simulink model "TIA"  (R2017b)
settings: Solver=VariableStepAuto  StartTime=0.0  StopTime=inf  RelTol=1e-3
undefined symbols (not defined in the file): sigbuilder_block
(part 1 of 2)
settings Model: PauseTimes=200  NumberOfSteps=10  Creator=matlab01  LastModifiedBy=matlab01

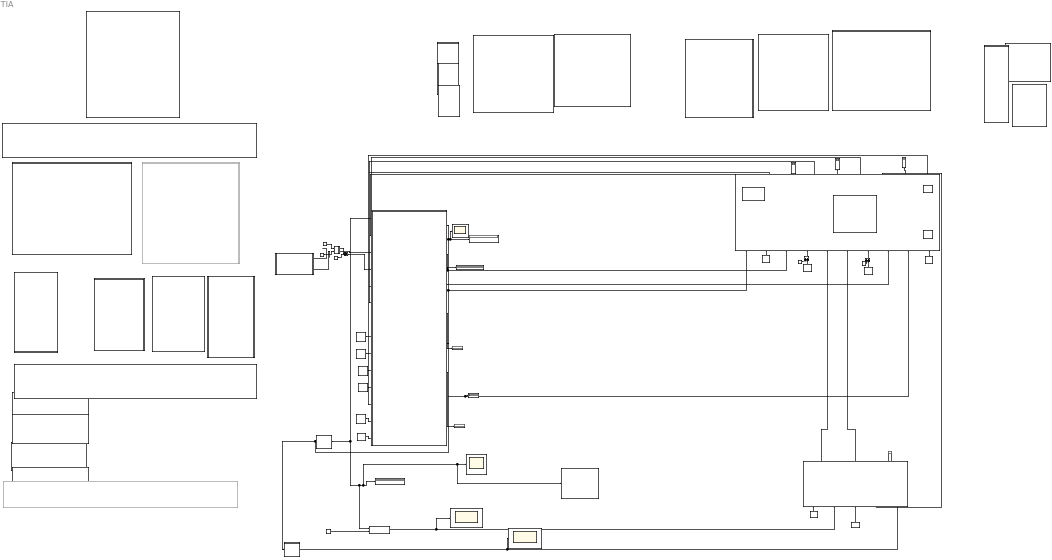
== system TIA ==
  note: Subsystem
  note: Subsystem
  note: User Input Board
  note: Subsystem
  note: Subsystem
  Add : Sum
  Add1 : Sum
  Add2 : Sum
  Bale Pass Sr : Constant  Value=0
  Bale Size Sr : Constant  Value=0
  Baler : Subsystem
  Baler Stopped : Subsystem  DialogController=hmiCreateDDGDialog  IsWebBlock=on  mask(MWDashboardBlock){webBlockId=380f0481-0464-4552-ac21-b39f29efcae4, webBlockType=lamp, ShowInLibBrowser=on, ShowInitialText=on, HMISrcModelName=TIA}
      mask prompts: webBlockType "WebBlock Type"; HMISrcModelName "Source Model"
      mask help: SimulinkHMI:dialogs:LampDialogDesc
      mask Help: helpview([docroot '/mapfiles/simulink.map'], 'hmi_lamp')
      mask Display:
      | if strcmp(get_param(bdroot(gcb),'BlockDiagramType'), 'library')
      |     image([(matlabroot) '/toolbox/simulink/hmi/icons/Lamp.png']);
      | end
  BalerCFG : DisplayBlock  WebBlockId=152  ModelName=TIA  LabelPosition=Hide  ShowInitialText=on  ShowFormattedStrings=off  Format=long  Alignment=Center
  CFG : Display
  Check Box : Checkbox  WebBlockId=154  ModelName=TIA  LabelPosition=Hide  ShowInitialText=off  Checked=on  Label=RearSr_1_Fail
  Check Box1 : Checkbox  WebBlockId=155  ModelName=TIA  LabelPosition=Hide  ShowInitialText=off  Checked=on  Label=RearSr_2_Fail
  Check Box2 : Checkbox  WebBlockId=156  ModelName=TIA  LabelPosition=Hide  ShowInitialText=off  Checked=off  Label=SpeedSr_Fail
  Check Box3 : Checkbox  WebBlockId=157  ModelName=TIA  LabelPosition=Hide  ShowInitialText=off  Checked=off  Label=FrontObstSr_Fail
  Constant : Constant  Value=2
  Constant1 : Constant  Value=2
  Constant2 : Constant  Value=2.7941176470588
  Display{,2,4..6} (5 alike) : Display
  Display3 : DisplayBlock  WebBlockId=163  ModelName=TIA  LabelPosition=Hide  ShowInitialText=on  ShowFormattedStrings=off  Format=long  Alignment=Center
  Display7 : DisplayBlock  WebBlockId=167  ModelName=TIA  LabelPosition=Hide  ShowInitialText=on  ShowFormattedStrings=off  Format=long  Alignment=Center
  DoorStatus : Display
  FinalSysSpeed : Scope
  Front Obstacle : Constant  Value=0
  FrontObstSr : Subsystem
  FrontObstSrFail : Constant  Value=0
  Gauge : Subsystem  DialogController=hmiCreateDDGDialog  IsWebBlock=on  mask(MWDashboardBlock){webBlockId=a8481909-2d34-4551-932e-729d5791eb58, webBlockType=circulargauge, ShowInLibBrowser=on, ShowInitialText=on, HMISrcModelName=TIA}
      mask prompts: webBlockId "WebBlock Id"; webBlockType "WebBlock Type"; HMISrcModelName "Source Model"
      mask help: SimulinkHMI:dialogs:CircularGaugeDialogDesc
      mask Help: helpview([docroot '/mapfiles/simulink.map'], 'hmi_gauge')
      mask Display:
      | if strcmp(get_param(bdroot(gcb),'BlockDiagramType'), 'library')
      |     image([(matlabroot) '/toolbox/simulink/hmi/icons/CircularGauge.png']);
      | end
  Knob : Subsystem  DialogController=hmiCreateDDGDialog  IsWebBlock=on  mask(MWDashboardBlock){webBlockId=44b2cfbf-7851-438f-9afd-65227a1c2716, webBlockType=continuousknob, ShowInLibBrowser=on, ShowInitialText=on, HMISrcModelName=TIA}
      mask prompts: webBlockId "WebBlock Id"; webBlockType "WebBlock Type"; HMISrcModelName "Source Model"
      mask help: SimulinkHMI:dialogs:ContinuousKnobDialogDesc
      mask Help: helpview([docroot '/mapfiles/simulink.map'], 'hmi_knob')
      mask Display:
      | if strcmp(get_param(bdroot(gcb),'BlockDiagramType'), 'library')
      |     image([(matlabroot) '/toolbox/simulink/hmi/icons/ContinuousKnob.png']);
      | end
  Knob1 : Subsystem  DialogController=hmiCreateDDGDialog  IsWebBlock=on  mask(MWDashboardBlock){webBlockId=555d5953-f540-48b0-b281-3241b1506ee0, webBlockType=continuousknob, ShowInLibBrowser=on, ShowInitialText=on, HMISrcModelName=TIA}
      mask prompts: webBlockId "WebBlock Id"; webBlockType "WebBlock Type"; HMISrcModelName "Source Model"
      mask help: SimulinkHMI:dialogs:ContinuousKnobDialogDesc
      mask Help: helpview([docroot '/mapfiles/simulink.map'], 'hmi_knob')
      mask Display:
      | if strcmp(get_param(bdroot(gcb),'BlockDiagramType'), 'library')
      |     image([(matlabroot) '/toolbox/simulink/hmi/icons/ContinuousKnob.png']);
      | end
  Lamp : Subsystem  DialogController=hmiCreateDDGDialog  IsWebBlock=on  mask(MWDashboardBlock){webBlockId=33d9c165-8687-4e0a-bfea-f4d86ec876ec, webBlockType=lamp, ShowInLibBrowser=on, ShowInitialText=on, HMISrcModelName=TIA}
      mask prompts: webBlockType "WebBlock Type"; HMISrcModelName "Source Model"
      mask help: SimulinkHMI:dialogs:LampDialogDesc
      mask Help: helpview([docroot '/mapfiles/simulink.map'], 'hmi_lamp')
      mask Display:
      | if strcmp(get_param(bdroot(gcb),'BlockDiagramType'), 'library')
      |     image([(matlabroot) '/toolbox/simulink/hmi/icons/Lamp.png']);
      | end
  Lamp1 : Subsystem  DialogController=hmiCreateDDGDialog  IsWebBlock=on  mask(MWDashboardBlock){webBlockId=c492ce9b-3337-4b76-9797-8f79f533d9ec, webBlockType=lamp, ShowInLibBrowser=on, ShowInitialText=on, HMISrcModelName=TIA}
      mask prompts: webBlockType "WebBlock Type"; HMISrcModelName "Source Model"
      mask help: SimulinkHMI:dialogs:LampDialogDesc
      mask Help: helpview([docroot '/mapfiles/simulink.map'], 'hmi_lamp')
      mask Display:
      | if strcmp(get_param(bdroot(gcb),'BlockDiagramType'), 'library')
      |     image([(matlabroot) '/toolbox/simulink/hmi/icons/Lamp.png']);
      | end
  Lamp2 : Subsystem  DialogController=hmiCreateDDGDialog  IsWebBlock=on  mask(MWDashboardBlock){webBlockId=4733d592-1260-498b-b033-10984541e09d, webBlockType=lamp, ShowInLibBrowser=on, ShowInitialText=on, HMISrcModelName=TIA}
      mask prompts: webBlockType "WebBlock Type"; HMISrcModelName "Source Model"
      mask help: SimulinkHMI:dialogs:LampDialogDesc
      mask Help: helpview([docroot '/mapfiles/simulink.map'], 'hmi_lamp')
      mask Display:
      | if strcmp(get_param(bdroot(gcb),'BlockDiagramType'), 'library')
      |     image([(matlabroot) '/toolbox/simulink/hmi/icons/Lamp.png']);
      | end
  Lamp3 : Subsystem  DialogController=hmiCreateDDGDialog  IsWebBlock=on  mask(MWDashboardBlock){webBlockId=748ac69b-6fb4-4b5c-9b27-9bec6aca2e03, webBlockType=lamp, ShowInLibBrowser=on, ShowInitialText=on, HMISrcModelName=TIA}
      mask prompts: webBlockType "WebBlock Type"; HMISrcModelName "Source Model"
      mask help: SimulinkHMI:dialogs:LampDialogDesc
      mask Help: helpview([docroot '/mapfiles/simulink.map'], 'hmi_lamp')
      mask Display:
      | if strcmp(get_param(bdroot(gcb),'BlockDiagramType'), 'library')
      |     image([(matlabroot) '/toolbox/simulink/hmi/icons/Lamp.png']);
      | end
  Lamp4 : Subsystem  DialogController=hmiCreateDDGDialog  IsWebBlock=on  mask(MWDashboardBlock){webBlockId=46aeaf17-ce96-4d45-93cb-a6cc3236d1da, webBlockType=lamp, ShowInLibBrowser=on, ShowInitialText=on, HMISrcModelName=TIA}
      mask prompts: webBlockType "WebBlock Type"; HMISrcModelName "Source Model"
      mask help: SimulinkHMI:dialogs:LampDialogDesc
      mask Help: helpview([docroot '/mapfiles/simulink.map'], 'hmi_lamp')
      mask Display:
      | if strcmp(get_param(bdroot(gcb),'BlockDiagramType'), 'library')
      |     image([(matlabroot) '/toolbox/simulink/hmi/icons/Lamp.png']);
      | end
  Lamp5 : Subsystem  DialogController=hmiCreateDDGDialog  IsWebBlock=on  mask(MWDashboardBlock){webBlockId=a14f3337-2fd1-43d0-b24a-5146b7c5b984, webBlockType=lamp, ShowInLibBrowser=on, ShowInitialText=on, HMISrcModelName=TIA}
      mask prompts: webBlockType "WebBlock Type"; HMISrcModelName "Source Model"
      mask help: SimulinkHMI:dialogs:LampDialogDesc
      mask Help: helpview([docroot '/mapfiles/simulink.map'], 'hmi_lamp')
      mask Display:
      | if strcmp(get_param(bdroot(gcb),'BlockDiagramType'), 'library')
      |     image([(matlabroot) '/toolbox/simulink/hmi/icons/Lamp.png']);
      | end
  Lamp6 : Subsystem  DialogController=hmiCreateDDGDialog  IsWebBlock=on  mask(MWDashboardBlock){webBlockId=0c8923f2-3b37-4230-bb87-17ac293e5df4, webBlockType=lamp, ShowInLibBrowser=on, ShowInitialText=on, HMISrcModelName=TIA}
      mask prompts: webBlockType "WebBlock Type"; HMISrcModelName "Source Model"
      mask help: SimulinkHMI:dialogs:LampDialogDesc
      mask Help: helpview([docroot '/mapfiles/simulink.map'], 'hmi_lamp')
      mask Display:
      | if strcmp(get_param(bdroot(gcb),'BlockDiagramType'), 'library')
      |     image([(matlabroot) '/toolbox/simulink/hmi/icons/Lamp.png']);
      | end
  Linear Gauge : Subsystem  DialogController=hmiCreateDDGDialog  IsWebBlock=on  mask(MWDashboardBlock){webBlockId=3991d636-6193-4a79-b88e-7eb4f4bb3acf, webBlockType=lineargauge, ShowInLibBrowser=on, ShowInitialText=on, HMISrcModelName=TIA}
      mask prompts: webBlockId "WebBlock Id"; webBlockType "WebBlock Type"; HMISrcModelName "Source Model"
      mask help: SimulinkHMI:dialogs:LinearGaugeDialogDesc
      mask Help: helpview([docroot '/mapfiles/simulink.map'], 'hmi_linear_gauge')
      mask Display:
      | if strcmp(get_param(bdroot(gcb),'BlockDiagramType'), 'library')
      |     image([(matlabroot) '/toolbox/simulink/hmi/icons/LinearGauge.png']);
      | end
  Need to stop : Display
  Product : Product
  RearDoor : Subsystem  DialogController=hmiCreateDDGDialog  IsWebBlock=on  mask(MWDashboardBlock){webBlockId=b538fc73-89be-495c-b7c3-b8c3e3397391, webBlockType=lamp, ShowInLibBrowser=on, ShowInitialText=on, HMISrcModelName=TIA}
      mask prompts: webBlockType "WebBlock Type"; HMISrcModelName "Source Model"
      mask help: SimulinkHMI:dialogs:LampDialogDesc
      mask Help: helpview([docroot '/mapfiles/simulink.map'], 'hmi_lamp')
      mask Display:
      | if strcmp(get_param(bdroot(gcb),'BlockDiagramType'), 'library')
      |     image([(matlabroot) '/toolbox/simulink/hmi/icons/Lamp.png']);
      | end
  RearObstSr : Subsystem  DialogController=hmiCreateDDGDialog  IsWebBlock=on  mask(MWDashboardBlock){webBlockId=2f04e0dc-cfdf-4b89-b502-650f31ce5fe2, webBlockType=rockerswitch, ShowInLibBrowser=on, ShowInitialText=on, HMISrcModelName=TIA}
      mask prompts: webBlockId "WebBlock Id"; webBlockType "WebBlock Type"; HMISrcModelName "Source Model"
      mask help: SimulinkHMI:dialogs:SwitchDialogDesc
      mask Help: helpview([docroot '/mapfiles/simulink.map'], 'hmi_rocker_switch')
      mask Display:
      | if strcmp(get_param(bdroot(gcb),'BlockDiagramType'), 'library')
      |     image([(matlabroot) '/toolbox/simulink/hmi/icons/RockerSwitch.png']);
      | end
  RearObstSr1 : Subsystem  DialogController=hmiCreateDDGDialog  IsWebBlock=on  mask(MWDashboardBlock){webBlockId=c64d6447-8e55-46e9-b568-5078a23053e9, webBlockType=rockerswitch, ShowInLibBrowser=on, ShowInitialText=on, HMISrcModelName=TIA}
      mask prompts: webBlockId "WebBlock Id"; webBlockType "WebBlock Type"; HMISrcModelName "Source Model"
      mask help: SimulinkHMI:dialogs:SwitchDialogDesc
      mask Help: helpview([docroot '/mapfiles/simulink.map'], 'hmi_rocker_switch')
      mask Display:
      | if strcmp(get_param(bdroot(gcb),'BlockDiagramType'), 'library')
      |     image([(matlabroot) '/toolbox/simulink/hmi/icons/RockerSwitch.png']);
      | end
  RearObstSr2 : Subsystem  DialogController=hmiCreateDDGDialog  IsWebBlock=on  mask(MWDashboardBlock){webBlockId=c4afeddd-f4a6-4f0c-9e01-adb611532535, webBlockType=rockerswitch, ShowInLibBrowser=on, ShowInitialText=on, HMISrcModelName=TIA}
      mask prompts: webBlockId "WebBlock Id"; webBlockType "WebBlock Type"; HMISrcModelName "Source Model"
      mask help: SimulinkHMI:dialogs:SwitchDialogDesc
      mask Help: helpview([docroot '/mapfiles/simulink.map'], 'hmi_rocker_switch')
      mask Display:
      | if strcmp(get_param(bdroot(gcb),'BlockDiagramType'), 'library')
      |     image([(matlabroot) '/toolbox/simulink/hmi/icons/RockerSwitch.png']);
      | end
  RearSr1 : Constant  Value=0
  RearSr2 : Constant  Value=0
  Rotary Switch : Subsystem  DialogController=hmiCreateDDGDialog  IsWebBlock=on  mask(MWDashboardBlock){webBlockId=4718e849-02b3-481c-8935-c4c34f11cecd, webBlockType=discreteknob, ShowInLibBrowser=on, ShowInitialText=on, HMISrcModelName=TIA}
      mask prompts: webBlockId "WebBlock Id"; webBlockType "WebBlock Type"; HMISrcModelName "Source Model"
      mask help: SimulinkHMI:dialogs:DiscreteKnobDialogDesc
      mask Help: helpview([docroot '/mapfiles/simulink.map'], 'hmi_rotary_switch')
      mask Display:
      | model = bdroot(gcb);
      | if strcmp(get_param(model,'BlockDiagramType'), 'library')
      |     image([(matlabroot) '/toolbox/simulink/hmi/icons/DiscreteKnob.png']);
      | end
  Rotary Switch1 : Subsystem  DialogController=hmiCreateDDGDialog  IsWebBlock=on  mask(MWDashboardBlock){webBlockId=f404cd82-44b9-4011-b588-6289506ab41c, webBlockType=discreteknob, ShowInLibBrowser=on, ShowInitialText=on, HMISrcModelName=TIA}
      mask prompts: webBlockId "WebBlock Id"; webBlockType "WebBlock Type"; HMISrcModelName "Source Model"
      mask help: SimulinkHMI:dialogs:DiscreteKnobDialogDesc
      mask Help: helpview([docroot '/mapfiles/simulink.map'], 'hmi_rotary_switch')
      mask Display:
      | model = bdroot(gcb);
      | if strcmp(get_param(model,'BlockDiagramType'), 'library')
      |     image([(matlabroot) '/toolbox/simulink/hmi/icons/DiscreteKnob.png']);
      | end
  Rotary Switch3 : Subsystem  DialogController=hmiCreateDDGDialog  IsWebBlock=on  mask(MWDashboardBlock){webBlockId=10fa69e3-8ad0-4a7e-b427-115ef8b6ee24, webBlockType=discreteknob, ShowInLibBrowser=on, ShowInitialText=on, HMISrcModelName=TIA}
      mask prompts: webBlockId "WebBlock Id"; webBlockType "WebBlock Type"; HMISrcModelName "Source Model"
      mask help: SimulinkHMI:dialogs:DiscreteKnobDialogDesc
      mask Help: helpview([docroot '/mapfiles/simulink.map'], 'hmi_rotary_switch')
      mask Display:
      | model = bdroot(gcb);
      | if strcmp(get_param(model,'BlockDiagramType'), 'library')
      |     image([(matlabroot) '/toolbox/simulink/hmi/icons/DiscreteKnob.png']);
      | end
  Scope : Scope
  SettedSpeed : Display
  Signal Builder : Subsystem  Tag=STV Subsys  LoadFcn=sigbuilder_block('load');  StartFcn=sigbuilder_block('start');  StopFcn=sigbuilder_block('stop');  ClipboardFcn=sigbuilder_block('clipboard');  mask(Sigbuilder block){tuvar=[0:10]}
      mask help: Simulink:masks:SigbuilderBlock_MD
      mask init:
      | if ~strcmp(get_param(bdroot(gcbh),'SimulationStatus'),'stopped') tuvar = sigbuilder_block('maskInit'); end
      settings: CopyFcn=sigbuilder_block('copy');  DeleteFcn=sigbuilder_block('delete');  ModelCloseFcn=sigbuilder_block('modelClose');  PreSaveFcn=sigbuilder_block('preSave');  PauseFcn=sigbuilder_block('pause');  ContinueFcn=sigbuilder_block('continue');  NameChangeFcn=sigbuilder_block('namechange');  OpenFcn=sigbuilder_block('open',[107.25 -48.75 897.75 700.5 ]);  CloseFcn=sigbuilder_block('close');
      mask Display: plot(0, 0, 100, 100,[2, 2, 32, 32, 2], [68, 8, 8, 68, 68],[32, 2], [38, 38], [32, 19, 2],[53, 60, 44], [32, 17, 17, 2],[16, 16, 31, 31]);txt = getActiveGroup(gcbh);text(2, 100, txt,'verticalAlignment', 'top');
  Slider : Subsystem  Commented=on  DialogController=hmiCreateDDGDialog  IsWebBlock=on  mask(MWDashboardBlock){webBlockId=15a6815c-0950-4bd8-89d9-de0febee8296, webBlockType=slider, ShowInLibBrowser=on, ShowInitialText=on, HMISrcModelName=TIA}
      mask prompts: webBlockId "WebBlock Id"; webBlockType "WebBlock Type"; HMISrcModelName "Source Model"
      mask help: SimulinkHMI:dialogs:SliderDialogDesc
      mask Help: helpview([docroot '/mapfiles/simulink.map'], 'hmi_slider')
      mask Display:
      | if strcmp(get_param(bdroot(gcb),'BlockDiagramType'), 'library')
      |     image([(matlabroot) '/toolbox/simulink/hmi/icons/Slider.png']);
      | end
  Slider1 : Subsystem  DialogController=hmiCreateDDGDialog  IsWebBlock=on  mask(MWDashboardBlock){webBlockId=472954f7-77f4-4c52-b158-1c9b312c99f5, webBlockType=slider, ShowInLibBrowser=on, ShowInitialText=on, HMISrcModelName=TIA}
      mask prompts: webBlockId "WebBlock Id"; webBlockType "WebBlock Type"; HMISrcModelName "Source Model"
      mask help: SimulinkHMI:dialogs:SliderDialogDesc
      mask Help: helpview([docroot '/mapfiles/simulink.map'], 'hmi_slider')
      mask Display:
      | if strcmp(get_param(bdroot(gcb),'BlockDiagramType'), 'library')
      |     image([(matlabroot) '/toolbox/simulink/hmi/icons/Slider.png']);
      | end
  SpSr1 : Scope
  SpSr1Fail : Constant
  SpSr2 : Scope
  "SpeedSr1 " : Subsystem
  SpeedSr2,3 : Subsystem
  SpeedUserInput : Constant  Value=1.1845603668526
  Steering Angle : Display
  SteeringUserInput : Constant  Value=-2.590329196644
  StopUserCMD : Constant  Value=0
  Swath  Area : Subsystem  Commented=on  DialogController=hmiCreateDDGDialog  IsWebBlock=on  mask(MathWorksWebBlock){webBlockId=664e3edd-25bd-4079-b9dd-da0d72c7846e, webBlockType=continuousknob, ShowInLibBrowser=on, ShowInitialText=on, HMISrcModelName=TIA}
      mask prompts: webBlockId "WebBlock Id"; webBlockType "WebBlock Type"; HMISrcModelName "Source Model"
      mask Help: helpview([docroot '/mapfiles/simulink.map'], 'hmi_knob')
      mask Display:
      | if strcmp(get_param(bdroot(gcb),'BlockDiagramType'), 'library')
      |     image([(matlabroot) '/toolbox/simulink/hmi/icons/ContinuousKnob.png']);
      | end
  Swath Area Value : Constant  Value=1.9663394927979
  SwathLocationSr : Constant  Value=2.5575447570332
  SwathScanner : Subsystem
  SysMode : Constant  Value=2
  To File1 : ToFile  SaveFormat=Timeseries
  Toggle Switch : Subsystem  DialogController=hmiCreateDDGDialog  IsWebBlock=on  mask(MWDashboardBlock){webBlockId=ef49c1b7-d3ac-49f4-96d4-aa01c0f2bdb4, webBlockType=toggleswitch, ShowInLibBrowser=on, ShowInitialText=on, HMISrcModelName=TIA}
      mask prompts: webBlockId "WebBlock Id"; webBlockType "WebBlock Type"; HMISrcModelName "Source Model"
      mask help: SimulinkHMI:dialogs:SwitchDialogDesc
      mask Help: helpview([docroot '/mapfiles/simulink.map'], 'hmi_toggle_switch')
      mask Display:
      | if strcmp(get_param(bdroot(gcb),'BlockDiagramType'), 'library')
      |     image([(matlabroot) '/toolbox/simulink/hmi/icons/ToggleSwitch.png']);
      | end
  Toggle Switch1 : Subsystem  DialogController=hmiCreateDDGDialog  IsWebBlock=on  mask(MWDashboardBlock){webBlockId=fecc03af-b420-4e0b-92e2-e06ee33ab186, webBlockType=toggleswitch, ShowInLibBrowser=on, ShowInitialText=on, HMISrcModelName=TIA}
      mask prompts: webBlockId "WebBlock Id"; webBlockType "WebBlock Type"; HMISrcModelName "Source Model"
      mask help: SimulinkHMI:dialogs:SwitchDialogDesc
      mask Help: helpview([docroot '/mapfiles/simulink.map'], 'hmi_toggle_switch')
      mask Display:
      | if strcmp(get_param(bdroot(gcb),'BlockDiagramType'), 'library')
      |     image([(matlabroot) '/toolbox/simulink/hmi/icons/ToggleSwitch.png']);
      | end
  Tractor : Subsystem
  User Present : Constant
  ValveUserCMD : Constant  Value=0
  frontObstSr : Subsystem  DialogController=hmiCreateDDGDialog  IsWebBlock=on  mask(MWDashboardBlock){webBlockId=dd25998f-ff44-4c86-97f2-224d2c2cc3c6, webBlockType=rockerswitch, ShowInLibBrowser=on, ShowInitialText=on, HMISrcModelName=TIA}
      mask prompts: webBlockId "WebBlock Id"; webBlockType "WebBlock Type"; HMISrcModelName "Source Model"
      mask help: SimulinkHMI:dialogs:SwitchDialogDesc
      mask Help: helpview([docroot '/mapfiles/simulink.map'], 'hmi_rocker_switch')
      mask Display:
      | if strcmp(get_param(bdroot(gcb),'BlockDiagramType'), 'library')
      |     image([(matlabroot) '/toolbox/simulink/hmi/icons/RockerSwitch.png']);
      | end
  wires:
  RearSr2/1 -> Add2/2
  Bale Size Sr/1 -> Baler/2(BaleSizeSr)
  Tractor/1(Speed) -> SpeedSr2,3/1(In1), "SpeedSr1 "/1(In1), Baler/1("settedSpeed "), SettedSpeed/1, Scope/1
  FrontObstSr/2(Out2) -> Tractor/3(In3)
  Baler/1(SetSpeedReq) -> Tractor/2(SpeedRequest)
  SwathScanner/3(CfgStatus) -> Display2/1
  Baler/3(StopSign) -> Display4/1
  Baler/7(RcfgCMD) -> SwathScanner/4(ReCfgCMD)
  Bale Pass Sr/1 -> Baler/10(BaleOutSr)
  Tractor/2(BrakiCMDCmd) -> Baler/3(StopComand), Display5/1
  User Present/1 -> Tractor/14(UserPresent)
  Product/1 -> SpSr1/1, SwathScanner/2(SpeedSr1)
  Baler/5(DoorSign) -> DoorStatus/1
  Baler/2("StopReq ") -> Tractor/5(StopReq)
  Baler/6(SetAngReq) -> Tractor/7(SetAngReq)
  Tractor/5("SysModeCmd ") -> Display6/1, Baler/9(ModeCngCMD)
  Signal Builder/1(FObstSr) -> ?
  Baler/4(DoorValveReq) -> Tractor/6(ValveReq)
  SteeringUserInput/1 -> Tractor/13(SteeringUserInput)
  RearSr1/1 -> Add1/2
  Swath Area Value/1 -> SwathScanner/1(In1)
  StopUserCMD/1 -> Tractor/9(StopUserInput)
  SpeedSr2,3/1(Out1) -> SpSr2/1, SwathScanner/5(SpeedSr2,3)
  SwathScanner/2(SwathLocation) -> Baler/6(SwathLocation)
  Tractor/4(SettedAng) -> Steering Angle/1
  Constant1/1 -> Add2/1
  SpSr1Fail/1 -> Product/2
  SwathLocationSr/1 -> SwathScanner/3(SwathLocationSr)
  SysMode/1 -> Tractor/8(SysMode)
  Tractor/6(BaleSizeLevel) -> Need to stop/1
  Baler/8(BalerCfg) -> CFG/1
  SpeedUserInput/1 -> Tractor/11(SpeedUserBedal)
  Baler/9(SysReconfigReq) -> Tractor/12("SysReconfigReq ")
  FrontObstSr/1(Out1) -> Add/1
  Tractor/3(Open/CloseCmd) -> Baler/8(RearDoorCmd)
  ValveUserCMD/1 -> Tractor/10(ValveUserInput)
  Add/1 -> Tractor/4(FrontObstSr)
  "SpeedSr1 "/1(Out1) -> Tractor/1(currentSpeed), Product/1, To File1/1, FinalSysSpeed/1, Display/1
  Constant/1 -> Add1/1
  FrontObstSrFail/1 -> Add/2
  Add1/1 -> Baler/4(RearObsSr1)
  Add2/1 -> Baler/7(RearObstSr2)
  SwathScanner/1(FlowRate) -> Baler/5(SwathVFlowRate)
  Signal Builder/2(Distance) -> ?
  Front Obstacle/1 -> FrontObstSr/1(In1)
  Constant2/1 -> FrontObstSr/2(In2)

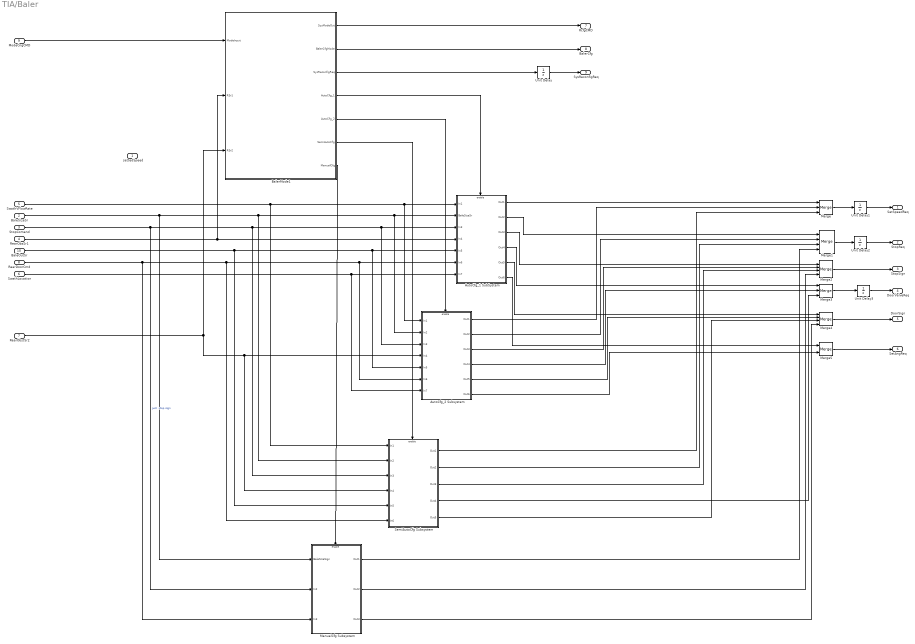
== system TIA/Baler ==
  "settedSpeed " : Inport
  BaleSizeSr : Inport  Port=2
  StopComand : Inport  Port=3
  RearObsSr1 : Inport  Port=4
  SwathVFlowRate : Inport  Port=5
  SwathLocation : Inport  Port=6
  RearObstSr2 : Inport  Port=7
  RearDoorCmd : Inport  Port=8
  ModeCngCMD : Inport  Port=9
  BaleOutSr : Inport  Port=10
  AutoCfg_1 SubSystem : Subsystem
  AutoCfg_2 Subsystem : Subsystem
  BalerMode1 : Stateflow chart  TreatAsAtomicUnit=on
  ManualCfg Subsystem : Subsystem
  Merge : Merge  Inputs=3
  Merge1 : Merge  Inputs=4
  Merge2 : Merge  Inputs=4
  Merge3 : Merge  Inputs=3
  Merge4 : Merge  Inputs=4
  Merge5 : Merge
  SemiAutoCfg Subsystem : Subsystem
  Unit Delay{,1..3} (4 alike) : UnitDelay  SampleTime=-1
  SetSpeedReq : Outport
  "StopReq " : Outport  Port=2
  StopSign : Outport  Port=3
  DoorValveReq : Outport  Port=4
  DoorSign : Outport  Port=5
  SetAngReq : Outport  Port=6
  RcfgCMD : Outport  Port=7
  BalerCfg : Outport  Port=8
  SysReconfigReq : Outport  Port=9
  wires:
  ModeCngCMD/1 -> BalerMode1/1(ModeInput)
  SwathVFlowRate/1 -> SemiAutoCfg Subsystem/1(In1), AutoCfg_2 Subsystem/1(In1), AutoCfg_1 SubSystem/1(In1)
  BaleSizeSr/1 -> SemiAutoCfg Subsystem/2(In2), AutoCfg_2 Subsystem/2(In2), AutoCfg_1 SubSystem/2(BaleSizeSr), ManualCfg Subsystem/1(BaleSizeSign)
  StopComand/1 -> ManualCfg Subsystem/2(In2), SemiAutoCfg Subsystem/3(In3), AutoCfg_2 Subsystem/3(In3), AutoCfg_1 SubSystem/3(In3)  "just  stop sign"
  RearObsSr1/1 -> BalerMode1/2(RSr1), AutoCfg_1 SubSystem/4(In4)
  BaleOutSr/1 -> SemiAutoCfg Subsystem/5(In5), AutoCfg_2 Subsystem/5(In5), AutoCfg_1 SubSystem/5(In5)
  RearDoorCmd/1 -> ManualCfg Subsystem/3(In3), SemiAutoCfg Subsystem/6(In6), AutoCfg_2 Subsystem/6(In6), AutoCfg_1 SubSystem/6(In6)
  SwathLocation/1 -> AutoCfg_2 Subsystem/7(In7), AutoCfg_1 SubSystem/7(In7)
  AutoCfg_1 SubSystem/3(Out3) -> Merge2/1
  AutoCfg_1 SubSystem/6(Out6) -> Merge5/1
  RearObstSr2/1 -> SemiAutoCfg Subsystem/4(In4), AutoCfg_2 Subsystem/4(In4), BalerMode1/3(RSr2)
  BalerMode1/1(SysModeOut) -> RcfgCMD/1
  BalerMode1/3(SysReconfigReq) -> Unit Delay/1
  Unit Delay/1 -> SysReconfigReq/1
  BalerMode1/4(AutoCfg_1) -> AutoCfg_1 SubSystem/Enable
  BalerMode1/5(AutoCfg_2) -> AutoCfg_2 Subsystem/Enable
  Merge/1 -> Unit Delay1/1
  Merge1/1 -> Unit Delay2/1
  Merge2/1 -> StopSign/1
  Merge3/1 -> Unit Delay3/1
  Merge4/1 -> DoorSign/1
  Merge5/1 -> SetAngReq/1
  AutoCfg_2 Subsystem/3(Out3) -> Merge2/2
  AutoCfg_1 SubSystem/5(Out5) -> Merge4/1
  AutoCfg_2 Subsystem/5(Out5) -> Merge4/2
  AutoCfg_2 Subsystem/6(Out6) -> Merge5/2
  AutoCfg_1 SubSystem/1(Out1) -> Merge/1
  AutoCfg_1 SubSystem/2(Out2) -> Merge1/1
  AutoCfg_1 SubSystem/4(Out4) -> Merge3/1
  AutoCfg_2 Subsystem/1(Out1) -> Merge/2
  AutoCfg_2 Subsystem/2(Out2) -> Merge1/2
  AutoCfg_2 Subsystem/4(Out4) -> Merge3/2
  Unit Delay2/1 -> "StopReq "/1
  Unit Delay3/1 -> DoorValveReq/1
  SemiAutoCfg Subsystem/1(Out1) -> Merge/3
  SemiAutoCfg Subsystem/2(Out2) -> Merge1/3
  SemiAutoCfg Subsystem/3(Out3) -> Merge2/3
  SemiAutoCfg Subsystem/4(Out4) -> Merge3/3
  SemiAutoCfg Subsystem/5(Out5) -> Merge4/3
  BalerMode1/6(SemiAutoCfg) -> SemiAutoCfg Subsystem/Enable
  BalerMode1/2(BalerCfgMode) -> BalerCfg/1
  ManualCfg Subsystem/1(Out1) -> Merge1/4
  BalerMode1/7(ManualCfg) -> ManualCfg Subsystem/Enable
  ManualCfg Subsystem/2(Out2) -> Merge2/4
  ManualCfg Subsystem/3(Out3) -> Merge4/4
  Unit Delay1/1 -> SetSpeedReq/1

== system TIA/Baler Stopped ==

== system TIA/FrontObstSr ==
  In1 : Inport
  In2 : Inport  Port=2
  Data Type Conversion : DataTypeConversion  OutDataTypeStr=boolean
  Out1 : Outport
  Out2 : Outport  Port=2
  wires:
  In1/1 -> Data Type Conversion/1
  Data Type Conversion/1 -> Out1/1
  In2/1 -> Out2/1

== system TIA/Gauge ==

== system TIA/Knob ==

== system TIA/Knob1 ==

== system TIA/Lamp ==

== system TIA/Lamp1 ==

== system TIA/Lamp2 ==

== system TIA/Lamp3 ==

== system TIA/Lamp4 ==

== system TIA/Lamp5 ==

== system TIA/Lamp6 ==

== system TIA/Linear Gauge ==

== system TIA/RearDoor ==

== system TIA/RearObstSr ==

== system TIA/RearObstSr1 ==

== system TIA/RearObstSr2 ==

== system TIA/Rotary Switch ==

== system TIA/Rotary Switch1 ==

== system TIA/Rotary Switch3 ==

== system TIA/Signal Builder ==
  Demux : Demux  Tag=STV Demux  Outputs=2
  FromWs : FromWorkspace  Tag=STV FromWs  VariableName=tuvar  SampleTime=0
      SigBuilderData=|
      | common.afterFinalStr = 'Extrapolate'
      | common.sampleTime = 0
      | dataSet.timeRange = [0 200]
      | dataSet.name = 'Group 1'
      | sbobj.Groups.Name = 'Group 1'
      | sbobj.Groups.Signals(1).Name = 'FObstSr'
      | sbobj.Groups.Signals(1).XData = [0 2 4 4 6 6 20 20 50 50 100 100 120 120 200]
      | sbobj.Groups.Signals(1).YData = [0 0 0 1 1 0 0 1 0.99 0 0 1 1 0 0]
      | sbobj.Groups.Signals(2).Name = 'Distance'
      | sbobj.Groups.Signals(2).XData = [0 4 7 50 100.2 110 120 120 139.8 140 200]
      | sbobj.Groups.Signals(2).YData = [4.98 5 4.3659043659 5 5 2.5 2 0 0 3.02 5.38]
      | sbobj.Groups.TimeRange = [0 200]
  FObstSr : Outport  Tag=STV Outport
  Distance : Outport  Tag=STV Outport  Port=2
  wires:
  Demux/1 -> FObstSr/1
  FromWs/1 -> Demux/1
  Demux/2 -> Distance/1

== system TIA/Slider ==

== system TIA/Slider1 ==

== system TIA/SpeedSr1  ==
  In1 : Inport
  Scope : Scope
  Signal Builder1 : Subsystem  Tag=STV Subsys  LoadFcn=sigbuilder_block('load');  StartFcn=sigbuilder_block('start');  StopFcn=sigbuilder_block('stop');  ClipboardFcn=sigbuilder_block('clipboard');  mask(Sigbuilder block){tuvar=[0:10]}
      mask help: Simulink:masks:SigbuilderBlock_MD
      mask init:
      | if ~strcmp(get_param(bdroot(gcbh),'SimulationStatus'),'stopped') tuvar = sigbuilder_block('maskInit'); end
      settings: CopyFcn=sigbuilder_block('copy');  DeleteFcn=sigbuilder_block('delete');  ModelCloseFcn=sigbuilder_block('modelClose');  PreSaveFcn=sigbuilder_block('preSave');  PauseFcn=sigbuilder_block('pause');  ContinueFcn=sigbuilder_block('continue');  NameChangeFcn=sigbuilder_block('namechange');  OpenFcn=sigbuilder_block('open',[438.75 215.25 544.5 355.5 ]);  CloseFcn=sigbuilder_block('close');
      mask Display: plot(0, 0, 100, 100,[2, 2, 32, 32, 2], [68, 8, 8, 68, 68],[32, 2], [38, 38], [32, 19, 2],[53, 60, 44], [32, 17, 17, 2],[16, 16, 31, 31]);txt = getActiveGroup(gcbh);text(2, 100, txt,'verticalAlignment', 'top');
  Switch : Switch
  Out1 : Outport
  wires:
  Signal Builder1/1(Signal 1) -> Switch/3, Switch/2
  In1/1 -> Switch/1, Scope/1
  Switch/1 -> Out1/1

== system TIA/SpeedSr2,3 ==
  In1 : Inport
  Signal Builder1 : Subsystem  Tag=STV Subsys  LoadFcn=sigbuilder_block('load');  StartFcn=sigbuilder_block('start');  StopFcn=sigbuilder_block('stop');  ClipboardFcn=sigbuilder_block('clipboard');  mask(Sigbuilder block){tuvar=[0:10]}
      mask help: Simulink:masks:SigbuilderBlock_MD
      mask init:
      | if ~strcmp(get_param(bdroot(gcbh),'SimulationStatus'),'stopped') tuvar = sigbuilder_block('maskInit'); end
      settings: CopyFcn=sigbuilder_block('copy');  DeleteFcn=sigbuilder_block('delete');  ModelCloseFcn=sigbuilder_block('modelClose');  PreSaveFcn=sigbuilder_block('preSave');  PauseFcn=sigbuilder_block('pause');  ContinueFcn=sigbuilder_block('continue');  NameChangeFcn=sigbuilder_block('namechange');  OpenFcn=sigbuilder_block('open',[438.75 215.25 544.5 355.5 ]);  CloseFcn=sigbuilder_block('close');
      mask Display: plot(0, 0, 100, 100,[2, 2, 32, 32, 2], [68, 8, 8, 68, 68],[32, 2], [38, 38], [32, 19, 2],[53, 60, 44], [32, 17, 17, 2],[16, 16, 31, 31]);txt = getActiveGroup(gcbh);text(2, 100, txt,'verticalAlignment', 'top');
  Switch : Switch
  Out1 : Outport
  wires:
  In1/1 -> Switch/1
  Switch/1 -> Out1/1
  Signal Builder1/1(Signal 1) -> Switch/2, Switch/3

== system TIA/Swath  Area ==

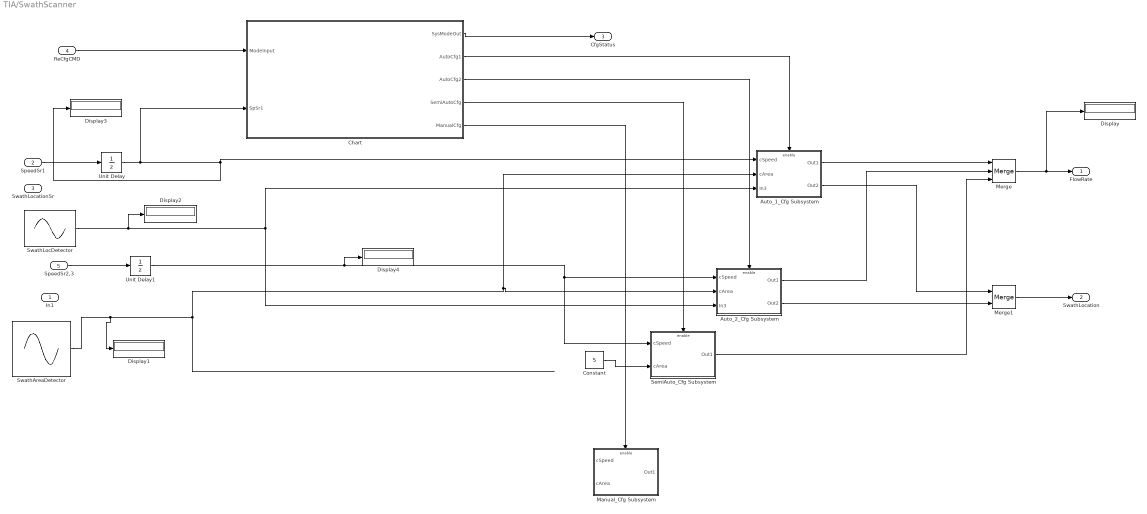
== system TIA/SwathScanner ==
  In1 : Inport
  SpeedSr1 : Inport  Port=2
  SwathLocationSr : Inport  Port=3
  ReCfgCMD : Inport  Port=4
  SpeedSr2,3 : Inport  Port=5
  Auto_1_Cfg Subsystem : Subsystem  TreatAsAtomicUnit=on
  Auto_2_Cfg Subsystem : Subsystem  TreatAsAtomicUnit=on
  Chart : Stateflow chart  TreatAsAtomicUnit=on
  Constant : Constant  Value=5
  Display{,1..4} (5 alike) : Display
  Manual_Cfg Subsystem : Subsystem  TreatAsAtomicUnit=on
  Merge : Merge  Inputs=3
  Merge1 : Merge
  SemiAuto_Cfg Subsystem : Subsystem  TreatAsAtomicUnit=on
  SwathAreaDetector : Sin  Amplitude=4  Bias=6  Frequency=0.001  SampleTime=0
  SwathLocDetector : Sin  Amplitude=4  Frequency=0.0003  SampleTime=0
  Unit Delay : UnitDelay  SampleTime=-1
  Unit Delay1 : UnitDelay  SampleTime=-1
  FlowRate : Outport
  SwathLocation : Outport  Port=2
  CfgStatus : Outport  Port=3
  wires:
  ReCfgCMD/1 -> Chart/1(ModeInput)
  Chart/1(SysModeOut) -> CfgStatus/1
  Auto_2_Cfg Subsystem/1(Out1) -> Merge/2
  SpeedSr2,3/1 -> Unit Delay1/1
  SwathAreaDetector/1 -> Display1/1, Auto_1_Cfg Subsystem/2(cArea), Auto_2_Cfg Subsystem/2(cArea)
  Auto_1_Cfg Subsystem/1(Out1) -> Merge/1
  Unit Delay/1 -> Chart/2(SpSr1), Display3/1, Auto_1_Cfg Subsystem/1(cSpeed)
  Merge/1 -> Display/1, FlowRate/1
  Unit Delay1/1 -> SemiAuto_Cfg Subsystem/1(cSpeed), Auto_2_Cfg Subsystem/1(cSpeed), Display4/1
  SpeedSr1/1 -> Unit Delay/1
  Chart/2(AutoCfg1) -> Auto_1_Cfg Subsystem/Enable
  Chart/3(AutoCfg2) -> Auto_2_Cfg Subsystem/Enable
  Chart/5(ManualCfg) -> Manual_Cfg Subsystem/Enable
  Chart/4(SemiAutoCfg) -> SemiAuto_Cfg Subsystem/Enable
  SwathLocDetector/1 -> Display2/1, Auto_1_Cfg Subsystem/3(In3), Auto_2_Cfg Subsystem/3(In3)
  Merge1/1 -> SwathLocation/1
  Auto_1_Cfg Subsystem/2(Out2) -> Merge1/1
  Auto_2_Cfg Subsystem/2(Out2) -> Merge1/2
  SemiAuto_Cfg Subsystem/1(Out1) -> Merge/3
  Constant/1 -> SemiAuto_Cfg Subsystem/2(cArea)

== system TIA/Toggle Switch ==

== system TIA/Toggle Switch1 ==

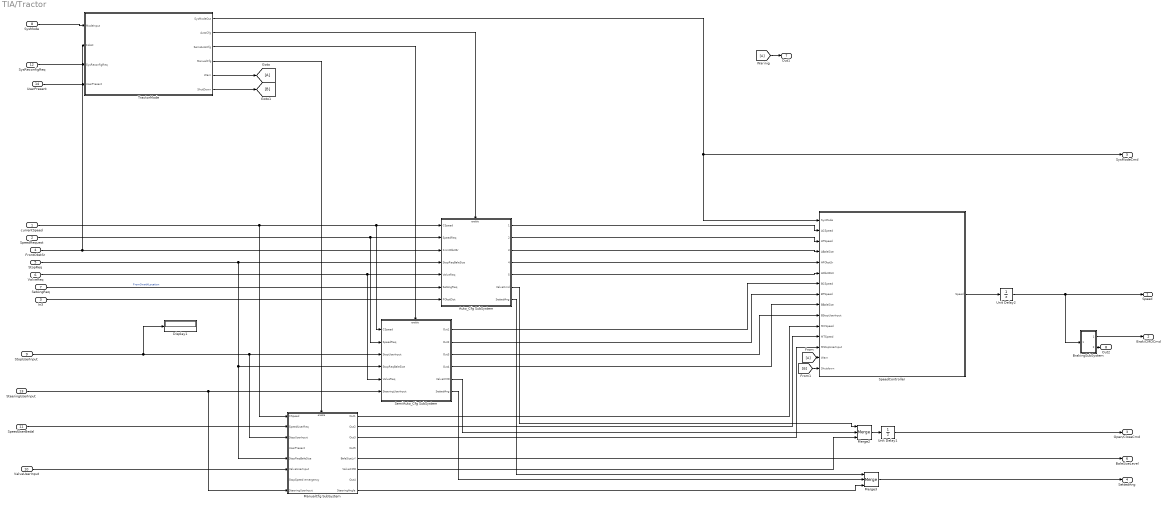
== system TIA/Tractor ==
  currentSpeed : Inport
  SpeedRequest : Inport  Port=2
  In3 : Inport  Port=3
  FrontObstSr : Inport  Port=4
  StopReq : Inport  Port=5
  ValveReq : Inport  Port=6
  SetAngReq : Inport  Port=7
  SysMode : Inport  Port=8
  StopUserInput : Inport  Port=9
  ValveUserInput : Inport  Port=10
  SpeedUserBedal : Inport  Port=11
  "SysReconfigReq " : Inport  Port=12
  SteeringUserInput : Inport  Port=13
  UserPresent : Inport  Port=14
  Auto_Cfg SubSystem : Subsystem
  BrakingSubSystem : Subsystem
  Display1 : Display
  ManualCfg SubSystem : Subsystem
  Merge2 : Merge  Inputs=3
  Merge3 : Merge  Inputs=3
  SemiAuto_Cfg SubSystem : Subsystem
  SpeedController : Stateflow chart  TreatAsAtomicUnit=on
  TractorMode : Stateflow chart  TreatAsAtomicUnit=on
  Unit Delay1 : UnitDelay  SampleTime=-1
  Unit Delay2 : UnitDelay  SampleTime=-1
  Speed : Outport
  BrakiCMDCmd : Outport  Port=2
  Open/CloseCmd : Outport  Port=3
  SettedAng : Outport  Port=4
  "SysModeCmd " : Outport  Port=5
  BaleSizeLevel : Outport  Port=6
  Out1 : Outport  Port=7
  Out2 : Outport  Port=8
  wires:
  FrontObstSr/1 -> TractorMode/2(Fobst), Auto_Cfg SubSystem/3(FrontObstSr)
  SetAngReq/1 -> Auto_Cfg SubSystem/6(SetAngReq)  "FromSwathLocation"
  SysMode/1 -> TractorMode/1(ModeInput)
  TractorMode/1(SysModeOut) -> "SysModeCmd "/1, SpeedController/1(SysMode)
  currentSpeed/1 -> SemiAuto_Cfg SubSystem/1(CSpeed), Auto_Cfg SubSystem/1(CSpeed), ManualCfg SubSystem/1(CSpeed)
  SpeedRequest/1 -> SemiAuto_Cfg SubSystem/2(SpeedReq), Auto_Cfg SubSystem/2(SpeedReq)
  StopReq/1 -> Auto_Cfg SubSystem/4(StopReqBaleSize), SemiAuto_Cfg SubSystem/4(StopReqBaleSize), ManualCfg SubSystem/5(StopReqBaleSize)
  ValveReq/1 -> SemiAuto_Cfg SubSystem/5(ValveReq), Auto_Cfg SubSystem/5(ValveReq)
  StopUserInput/1 -> Display1/1, SemiAuto_Cfg SubSystem/3(StopUserInput), ManualCfg SubSystem/3(StopUserInput)
  TractorMode/2(AutoCfg) -> Auto_Cfg SubSystem/Enable
  TractorMode/3(SemiAutoCfg) -> SemiAuto_Cfg SubSystem/Enable
  SemiAuto_Cfg SubSystem/5(ValveCMD) -> Merge2/2
  Merge2/1 -> Unit Delay1/1
  Auto_Cfg SubSystem/6(ValveCmd) -> Merge2/1
  TractorMode/4(ManualCfg) -> ManualCfg SubSystem/Enable
  SpeedUserBedal/1 -> ManualCfg SubSystem/2(SpeedUserReq)
  ValveUserInput/1 -> ManualCfg SubSystem/6(ValveUserInput)
  "SysReconfigReq "/1 -> TractorMode/3(SysReconfigReq)
  SteeringUserInput/1 -> ManualCfg SubSystem/8(SteeringUserInput), SemiAuto_Cfg SubSystem/6(SteeringUserInput)
  ManualCfg SubSystem/6(ValveCMD) -> Merge2/3
  Merge3/1 -> SettedAng/1
  Auto_Cfg SubSystem/7(SettedAng) -> Merge3/1
  SemiAuto_Cfg SubSystem/6(SettedAng) -> Merge3/2
  ManualCfg SubSystem/8(SteeringAngle) -> Merge3/3
  Unit Delay1/1 -> Open/CloseCmd/1
  ManualCfg SubSystem/5(BaleSizeLvl) -> BaleSizeLevel/1
  UserPresent/1 -> TractorMode/4(UserPresent)
  In3/1 -> Auto_Cfg SubSystem/7(FObstDist)
  Auto_Cfg SubSystem/1(1) -> SpeedController/2(ACSpeed)
  Auto_Cfg SubSystem/2(2) -> SpeedController/3(ATSpeed)
  Auto_Cfg SubSystem/3(3) -> SpeedController/4(ABaleSize)
  Auto_Cfg SubSystem/4(4) -> SpeedController/5(AFObstSr)
  Auto_Cfg SubSystem/5(5) -> SpeedController/6(AObstDist)
  SemiAuto_Cfg SubSystem/1(Out1) -> SpeedController/7(BCSpeed)
  SemiAuto_Cfg SubSystem/2(Out2) -> SpeedController/8(BTSpeed)
  SemiAuto_Cfg SubSystem/3(Out3) -> SpeedController/10(BStopUserInput)
  SemiAuto_Cfg SubSystem/4(Out4) -> SpeedController/9(BBaleSize)
  ManualCfg SubSystem/1(Out1) -> SpeedController/11(MCSpeed)
  ManualCfg SubSystem/2(Out2) -> SpeedController/12(MTSpeed)
  ManualCfg SubSystem/3(Out3) -> SpeedController/13(MStopUserInput)
  SpeedController/1(Speed) -> Unit Delay2/1
  Unit Delay2/1 -> BrakingSubSystem/1(In1), Speed/1
  TractorMode/5(" Warn") -> [A]
  [A] -> SpeedController/14(Warn)
  TractorMode/6(" ShutDown") -> [B]
  [B] -> SpeedController/15(Shutdown)
  [A] -> Out1/1
  BrakingSubSystem/1(Out1) -> BrakiCMDCmd/1
  BrakingSubSystem/2(Out2) -> Out2/1

== system TIA/frontObstSr ==

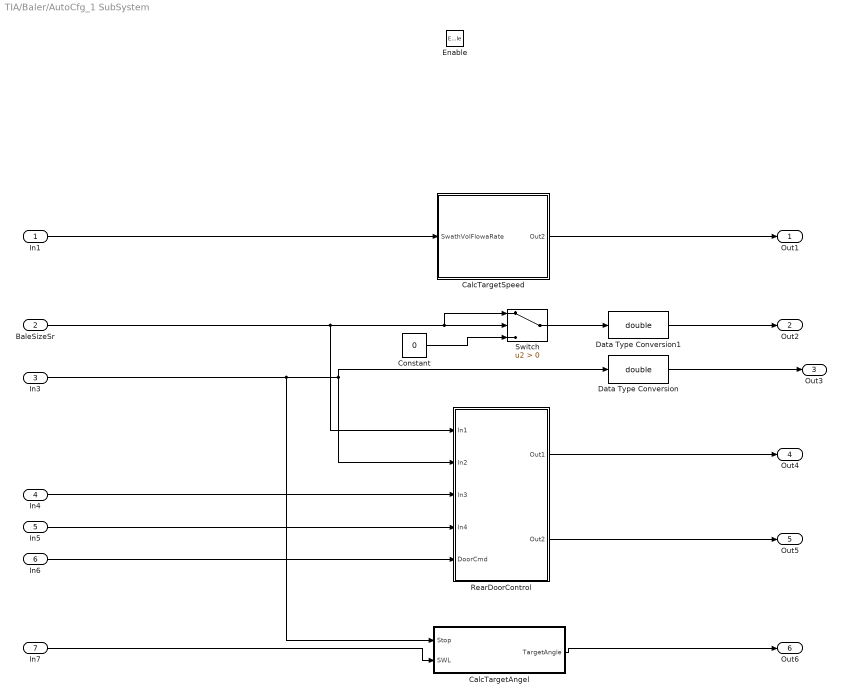
== system TIA/Baler/AutoCfg_1 SubSystem ==
  In1 : Inport
  BaleSizeSr : Inport  Port=2
  In3 : Inport  Port=3
  In4 : Inport  Port=4
  In5 : Inport  Port=5
  In6 : Inport  Port=6
  In7 : Inport  Port=7
  Enable : EnablePort
  CalcTargetAngel : MATLAB Function  TreatAsAtomicUnit=on
  CalcTargetSpeed : Subsystem
  Constant : Constant  Value=0
  Data Type Conversion : DataTypeConversion  OutDataTypeStr=double
  Data Type Conversion1 : DataTypeConversion  OutDataTypeStr=double
  RearDoorControl : Subsystem
  Switch : Switch  Criteria=u2 > Threshold
  Out1 : Outport
  Out2 : Outport  Port=2
  Out3 : Outport  Port=3  OutDataTypeStr=double
  Out4 : Outport  Port=4
  Out5 : Outport  Port=5
  Out6 : Outport  Port=6
  wires:
  CalcTargetSpeed/1(Out2) -> Out1/1
  In1/1 -> CalcTargetSpeed/1(SwathVolFlowaRate)
  Switch/1 -> Data Type Conversion1/1
  In6/1 -> RearDoorControl/5(DoorCmd)
  In3/1 -> CalcTargetAngel/1(Stop), Data Type Conversion/1, RearDoorControl/2(In2)
  RearDoorControl/1(Out1) -> Out4/1
  In7/1 -> CalcTargetAngel/2(SWL)
  In4/1 -> RearDoorControl/3(In3)
  In5/1 -> RearDoorControl/4(In4)
  BaleSizeSr/1 -> RearDoorControl/1(In1), Switch/1, Switch/2
  RearDoorControl/2(Out2) -> Out5/1
  CalcTargetAngel/1(TargetAngle) -> Out6/1
  Constant/1 -> Switch/3
  Data Type Conversion/1 -> Out3/1
  Data Type Conversion1/1 -> Out2/1

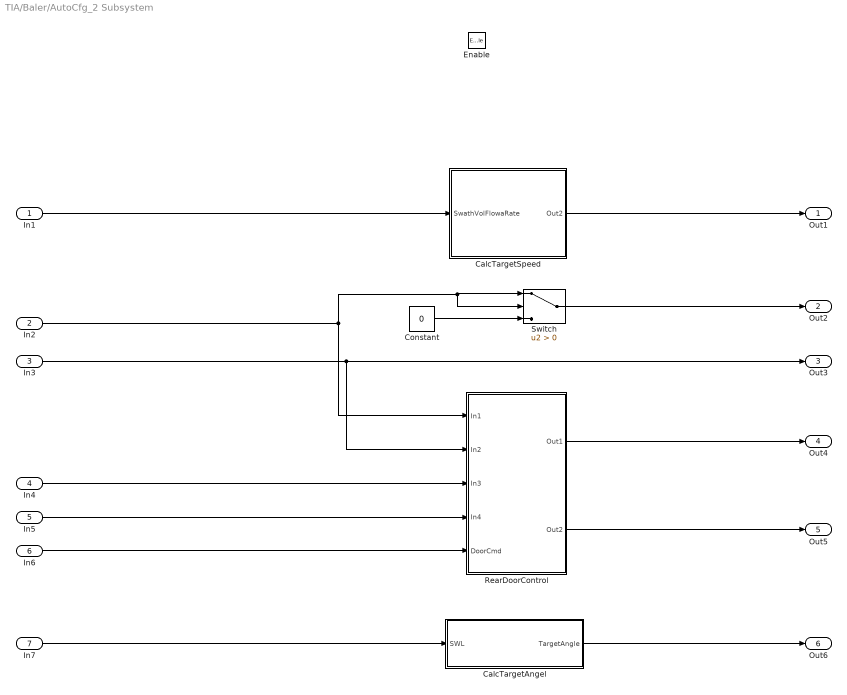
== system TIA/Baler/AutoCfg_2 Subsystem ==
  In1 : Inport
  In2 : Inport  Port=2
  In3 : Inport  Port=3
  In4 : Inport  Port=4
  In5 : Inport  Port=5
  In6 : Inport  Port=6
  In7 : Inport  Port=7
  Enable : EnablePort
  CalcTargetAngel : MATLAB Function  TreatAsAtomicUnit=on
  CalcTargetSpeed : Subsystem
  Constant : Constant  Value=0
  RearDoorControl : Subsystem
  Switch : Switch  Criteria=u2 > Threshold
  Out1 : Outport
  Out2 : Outport  Port=2
  Out3 : Outport  Port=3
  Out4 : Outport  Port=4
  Out5 : Outport  Port=5
  Out6 : Outport  Port=6
  wires:
  Constant/1 -> Switch/3
  CalcTargetAngel/1(TargetAngle) -> Out6/1
  RearDoorControl/2(Out2) -> Out5/1
  In2/1 -> RearDoorControl/1(In1), Switch/1, Switch/2
  In5/1 -> RearDoorControl/4(In4)
  In4/1 -> RearDoorControl/3(In3)
  In7/1 -> CalcTargetAngel/1(SWL)
  RearDoorControl/1(Out1) -> Out4/1
  In3/1 -> Out3/1, RearDoorControl/2(In2)
  In6/1 -> RearDoorControl/5(DoorCmd)
  Switch/1 -> Out2/1
  In1/1 -> CalcTargetSpeed/1(SwathVolFlowaRate)
  CalcTargetSpeed/1(Out2) -> Out1/1

== system TIA/Baler/ManualCfg Subsystem ==
  BaleSizeSign : Inport
  In2 : Inport  Port=2
  In3 : Inport  Port=3
  Enable : EnablePort
  Out1 : Outport
  Out2 : Outport  Port=2
  Out3 : Outport  Port=3
  wires:
  BaleSizeSign/1 -> Out1/1
  In2/1 -> Out2/1
  In3/1 -> Out3/1

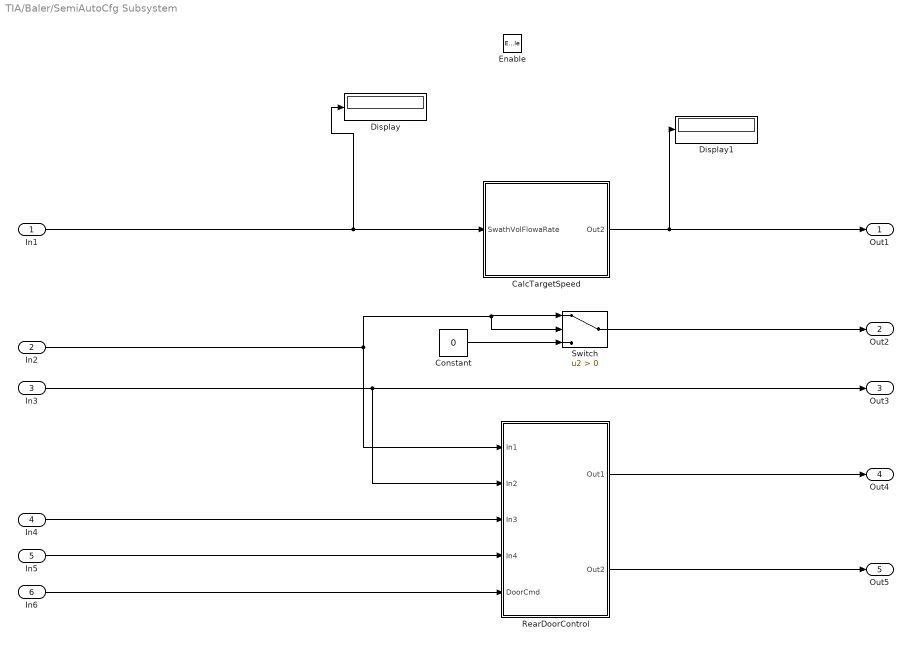
== system TIA/Baler/SemiAutoCfg Subsystem ==
  In1 : Inport
  In2 : Inport  Port=2
  In3 : Inport  Port=3
  In4 : Inport  Port=4
  In5 : Inport  Port=5
  In6 : Inport  Port=6
  Enable : EnablePort
  CalcTargetSpeed : Subsystem
  Constant : Constant  Value=0
  Display : Display
  Display1 : Display
  RearDoorControl : Subsystem
  Switch : Switch  Criteria=u2 > Threshold
  Out1 : Outport
  Out2 : Outport  Port=2
  Out3 : Outport  Port=3
  Out4 : Outport  Port=4
  Out5 : Outport  Port=5
  wires:
  CalcTargetSpeed/1(Out2) -> Display1/1, Out1/1
  In1/1 -> Display/1, CalcTargetSpeed/1(SwathVolFlowaRate)
  Switch/1 -> Out2/1
  In6/1 -> RearDoorControl/5(DoorCmd)
  In3/1 -> Out3/1, RearDoorControl/2(In2)
  RearDoorControl/1(Out1) -> Out4/1
  In4/1 -> RearDoorControl/3(In3)
  In5/1 -> RearDoorControl/4(In4)
  In2/1 -> Switch/2, Switch/1, RearDoorControl/1(In1)
  RearDoorControl/2(Out2) -> Out5/1
  Constant/1 -> Switch/3

== system TIA/SpeedSr1 /Signal Builder1 ==
  Demux : Demux  Tag=STV Demux  Outputs=1
  FromWs : FromWorkspace  Tag=STV FromWs  VariableName=tuvar  SampleTime=0
      SigBuilderData=|
      | common.afterFinalStr = 'Extrapolate'
      | common.sampleTime = 0
      | dataSet.timeRange = [0 20]
      | dataSet.name = 'Group 1'
      | sbobj.Groups.Name = 'Group 1'
      | sbobj.Groups.Signals.Name = 'Signal 1'
      | sbobj.Groups.Signals.XData = [0 4 6 8 10 20]
      | sbobj.Groups.Signals.YData = [0 4 5.95 10 10 10]
      | sbobj.Groups.TimeRange = [0 20]
  Signal 1 : Outport  Tag=STV Outport
  wires:
  Demux/1 -> Signal 1/1
  FromWs/1 -> Demux/1

== system TIA/SpeedSr2,3/Signal Builder1 ==
  Demux : Demux  Tag=STV Demux  Outputs=1
  FromWs : FromWorkspace  Tag=STV FromWs  VariableName=tuvar  SampleTime=0
      SigBuilderData=|
      | common.afterFinalStr = 'Extrapolate'
      | common.sampleTime = 0
      | dataSet.timeRange = [0 20]
      | dataSet.name = 'Group 1'
      | sbobj.Groups.Name = 'Group 1'
      | sbobj.Groups.Signals.Name = 'Signal 1'
      | sbobj.Groups.Signals.XData = [0 4 6 8 10 20]
      | sbobj.Groups.Signals.YData = [0 4 5.95 10 10 10]
      | sbobj.Groups.TimeRange = [0 20]
  Signal 1 : Outport  Tag=STV Outport
  wires:
  FromWs/1 -> Demux/1
  Demux/1 -> Signal 1/1

== system TIA/SwathScanner/Auto_1_Cfg Subsystem ==
  cSpeed : Inport
  cArea : Inport  Port=2
  In3 : Inport  Port=3
  Enable : EnablePort  StatesWhenEnabling=reset
  CalcVolFlowRate 1 : Subsystem
  Out1 : Outport
  Out2 : Outport  Port=2
  wires:
  cSpeed/1 -> CalcVolFlowRate 1/1(CurrentSpeed)
  CalcVolFlowRate 1/1(Out1) -> Out1/1
  cArea/1 -> CalcVolFlowRate 1/2(SwathArea)
  In3/1 -> Out2/1

== system TIA/SwathScanner/Auto_2_Cfg Subsystem ==
  cSpeed : Inport
  cArea : Inport  Port=2
  In3 : Inport  Port=3
  Enable : EnablePort
  CalcVolFlowRate 1 : Subsystem
  Out1 : Outport
  Out2 : Outport  Port=2
  wires:
  cArea/1 -> CalcVolFlowRate 1/2(SwathArea)
  CalcVolFlowRate 1/1(Out1) -> Out1/1
  cSpeed/1 -> CalcVolFlowRate 1/1(CurrentSpeed)
  In3/1 -> Out2/1

== system TIA/SwathScanner/Manual_Cfg Subsystem ==
  cSpeed : Inport
  cArea : Inport  Port=2
  Enable : EnablePort
  CalcVolFlowRate 1 : Subsystem
  Out1 : Outport
  wires:
  cSpeed/1 -> CalcVolFlowRate 1/1(CurrentSpeed)
  CalcVolFlowRate 1/1(Out1) -> Out1/1
  cArea/1 -> CalcVolFlowRate 1/2(SwathArea)

== system TIA/SwathScanner/SemiAuto_Cfg Subsystem ==
  cSpeed : Inport
  cArea : Inport  Port=2
  Enable : EnablePort
  CalcVolFlowRate 1 : Subsystem
  Out1 : Outport
  wires:
  cSpeed/1 -> CalcVolFlowRate 1/1(CurrentSpeed)
  CalcVolFlowRate 1/1(Out1) -> Out1/1
  cArea/1 -> CalcVolFlowRate 1/2(SwathArea)

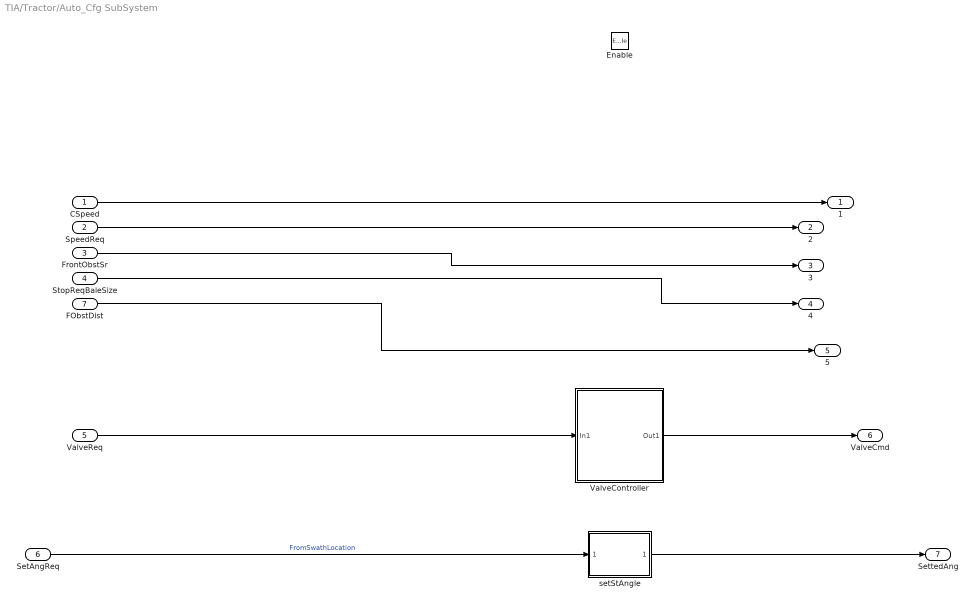
== system TIA/Tractor/Auto_Cfg SubSystem ==
  CSpeed : Inport
  SpeedReq : Inport  Port=2
  FrontObstSr : Inport  Port=3
  StopReqBaleSize : Inport  Port=4
  ValveReq : Inport  Port=5
  SetAngReq : Inport  Port=6
  FObstDist : Inport  Port=7
  Enable : EnablePort
  ValveController : Subsystem
  setStAngle : MATLAB Function  TreatAsAtomicUnit=on
  1 : Outport
  2 : Outport  Port=2
  3 : Outport  Port=3
  4 : Outport  Port=4
  5 : Outport  Port=5
  ValveCmd : Outport  Port=6
  SettedAng : Outport  Port=7
  wires:
  SpeedReq/1 -> 2/1
  ValveController/1(Out1) -> ValveCmd/1
  ValveReq/1 -> ValveController/1(In1)
  StopReqBaleSize/1 -> 4/1
  CSpeed/1 -> 1/1
  SetAngReq/1 -> setStAngle/1(TAngle)  "FromSwathLocation"
  setStAngle/1(CAngle) -> SettedAng/1
  FObstDist/1 -> 5/1
  FrontObstSr/1 -> 3/1

== system TIA/Tractor/BrakingSubSystem ==
  In1 : Inport
  Constant : Constant  Value=0
  Constant1 : Constant
  Constant2 : Constant  Value=2
  Switch : Switch  Criteria=u2 ~= 0
  Switch2 : Switch  Criteria=u2 ~= 0  Threshold=2
  Unit Delay : UnitDelay  SampleTime=-1
  Out1 : Outport
  Out2 : Outport  Port=2
  wires:
  Constant2/1 -> Switch/1
  In1/1 -> Switch2/2
  Unit Delay/1 -> Switch/3
  Constant1/1 -> Switch2/3
  Constant/1 -> Switch2/1
  [B] -> Out2/1, Switch/2
  Switch/1 -> Out1/1
  Switch2/1 -> Unit Delay/1

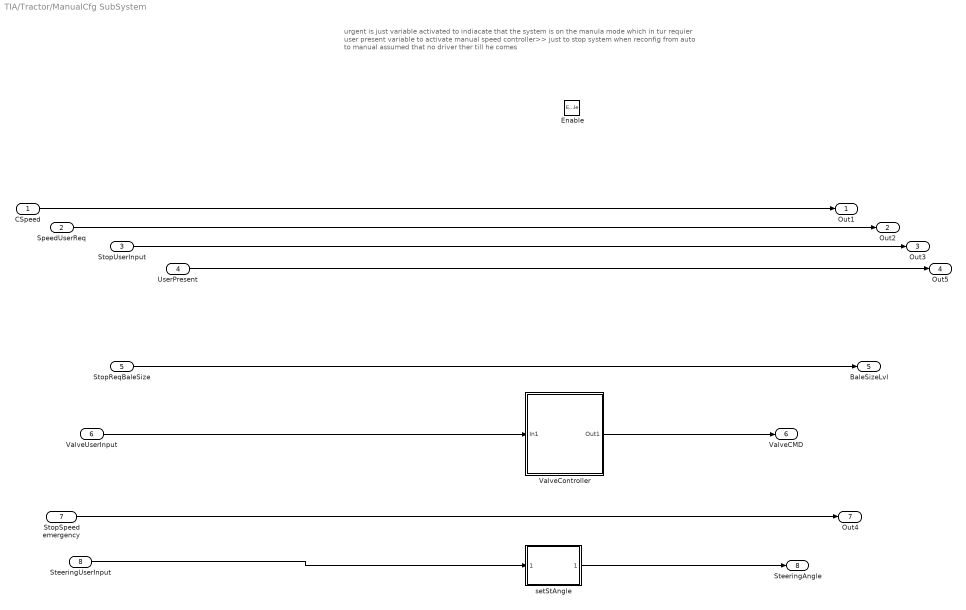
== system TIA/Tractor/ManualCfg SubSystem ==
  note: urgent is just variable activated to indiacate that the system is on the manula mode which in tur requier user present variable to activate manual speed controller>> just to stop system when reconfig from auto to manual assumed that no driver ther till he comes
  CSpeed : Inport
  SpeedUserReq : Inport  Port=2
  StopUserInput : Inport  Port=3
  UserPresent : Inport  Port=4
  StopReqBaleSize : Inport  Port=5
  ValveUserInput : Inport  Port=6
  StopSpeed emergency : Inport  Port=7
  SteeringUserInput : Inport  Port=8
  Enable : EnablePort
  ValveController : Subsystem
  setStAngle : MATLAB Function  TreatAsAtomicUnit=on
  Out1 : Outport
  Out2 : Outport  Port=2
  Out3 : Outport  Port=3
  Out5 : Outport  Port=4
  BaleSizeLvl : Outport  Port=5
  ValveCMD : Outport  Port=6
  Out4 : Outport  Port=7
  SteeringAngle : Outport  Port=8
  wires:
  ValveController/1(Out1) -> ValveCMD/1
  ValveUserInput/1 -> ValveController/1(In1)
  SteeringUserInput/1 -> setStAngle/1(TAngle)
  setStAngle/1(CAngle) -> SteeringAngle/1
  StopReqBaleSize/1 -> BaleSizeLvl/1
  CSpeed/1 -> Out1/1
  SpeedUserReq/1 -> Out2/1
  StopUserInput/1 -> Out3/1
  StopSpeed emergency/1 -> Out4/1
  UserPresent/1 -> Out5/1

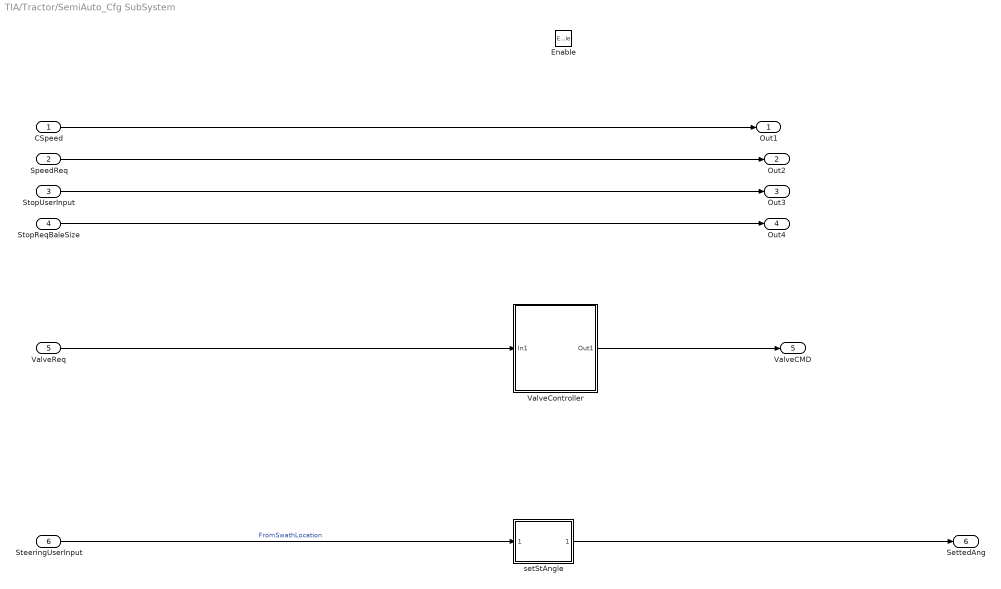
== system TIA/Tractor/SemiAuto_Cfg SubSystem ==
  CSpeed : Inport
  SpeedReq : Inport  Port=2
  StopUserInput : Inport  Port=3
  StopReqBaleSize : Inport  Port=4
  ValveReq : Inport  Port=5
  SteeringUserInput : Inport  Port=6
  Enable : EnablePort
  ValveController : Subsystem
  setStAngle : MATLAB Function  TreatAsAtomicUnit=on
  Out1 : Outport
  Out2 : Outport  Port=2
  Out3 : Outport  Port=3
  Out4 : Outport  Port=4
  ValveCMD : Outport  Port=5
  SettedAng : Outport  Port=6
  wires:
  ValveReq/1 -> ValveController/1(In1)
  ValveController/1(Out1) -> ValveCMD/1
  SteeringUserInput/1 -> setStAngle/1(TAngle)  "FromSwathLocation"
  setStAngle/1(CAngle) -> SettedAng/1
  CSpeed/1 -> Out1/1
  SpeedReq/1 -> Out2/1
  StopUserInput/1 -> Out3/1
  StopReqBaleSize/1 -> Out4/1

== system TIA/Baler/AutoCfg_1 SubSystem/CalcTargetSpeed ==
  SwathVolFlowaRate : Inport
  MATLAB Function : MATLAB Function  TreatAsAtomicUnit=on
  Out2 : Outport
  wires:
  SwathVolFlowaRate/1 -> MATLAB Function/1(u)
  MATLAB Function/1(TargetSpeed) -> Out2/1

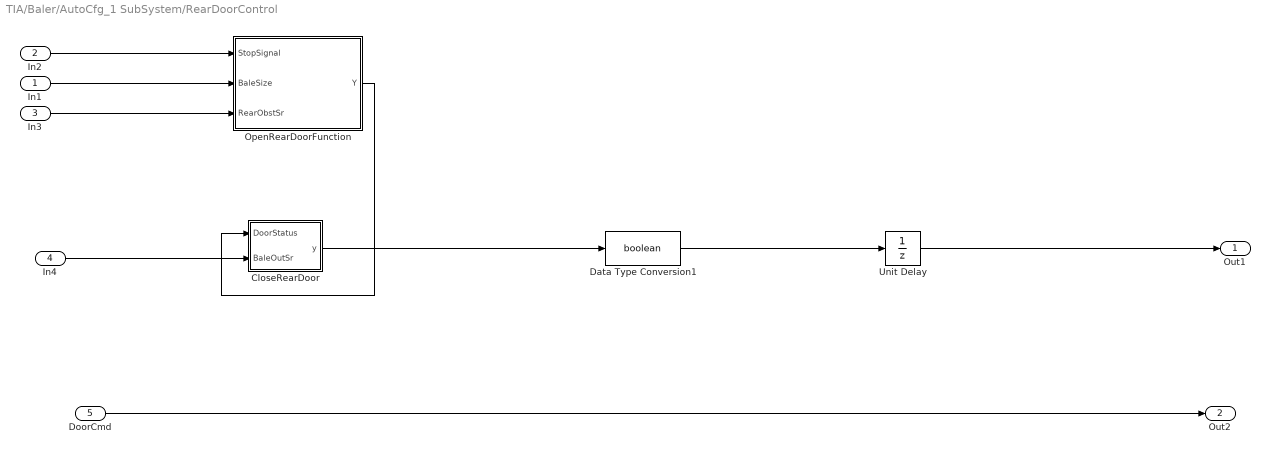
== system TIA/Baler/AutoCfg_1 SubSystem/RearDoorControl ==
  In1 : Inport
  In2 : Inport  Port=2
  In3 : Inport  Port=3
  In4 : Inport  Port=4
  DoorCmd : Inport  Port=5
  CloseRearDoor : MATLAB Function  TreatAsAtomicUnit=on
  Data Type Conversion1 : DataTypeConversion  OutDataTypeStr=boolean
  OpenRearDoorFunction : MATLAB Function  TreatAsAtomicUnit=on
  Unit Delay : UnitDelay  SampleTime=-1
  Out1 : Outport
  Out2 : Outport  Port=2
  wires:
  CloseRearDoor/1(y) -> Data Type Conversion1/1
  In3/1 -> OpenRearDoorFunction/3(RearObstSr)
  OpenRearDoorFunction/1(Y) -> CloseRearDoor/1(DoorStatus)
  Data Type Conversion1/1 -> Unit Delay/1
  In1/1 -> OpenRearDoorFunction/2(BaleSize)
  In2/1 -> OpenRearDoorFunction/1(StopSignal)
  In4/1 -> CloseRearDoor/2(BaleOutSr)
  DoorCmd/1 -> Out2/1
  Unit Delay/1 -> Out1/1

== system TIA/Baler/AutoCfg_2 Subsystem/CalcTargetSpeed ==
  SwathVolFlowaRate : Inport
  MATLAB Function : MATLAB Function  TreatAsAtomicUnit=on
  Out2 : Outport
  wires:
  MATLAB Function/1(TargetSpeed) -> Out2/1
  SwathVolFlowaRate/1 -> MATLAB Function/1(u)

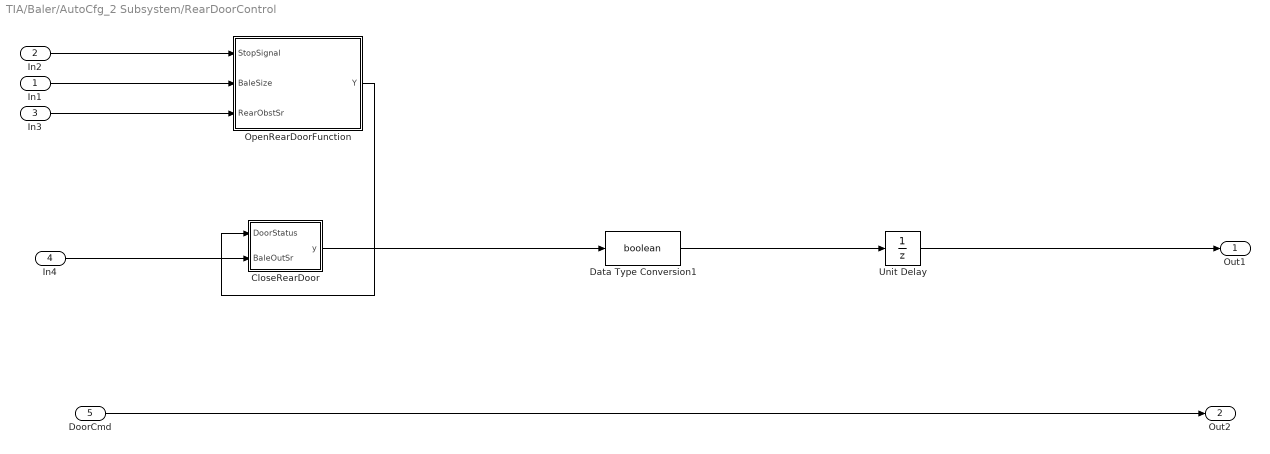
== system TIA/Baler/AutoCfg_2 Subsystem/RearDoorControl ==
  In1 : Inport
  In2 : Inport  Port=2
  In3 : Inport  Port=3
  In4 : Inport  Port=4
  DoorCmd : Inport  Port=5
  CloseRearDoor : MATLAB Function  TreatAsAtomicUnit=on
  Data Type Conversion1 : DataTypeConversion  OutDataTypeStr=boolean
  OpenRearDoorFunction : MATLAB Function  TreatAsAtomicUnit=on
  Unit Delay : UnitDelay  SampleTime=-1
  Out1 : Outport
  Out2 : Outport  Port=2
  wires:
  Unit Delay/1 -> Out1/1
  DoorCmd/1 -> Out2/1
  In4/1 -> CloseRearDoor/2(BaleOutSr)
  In2/1 -> OpenRearDoorFunction/1(StopSignal)
  In1/1 -> OpenRearDoorFunction/2(BaleSize)
  Data Type Conversion1/1 -> Unit Delay/1
  OpenRearDoorFunction/1(Y) -> CloseRearDoor/1(DoorStatus)
  In3/1 -> OpenRearDoorFunction/3(RearObstSr)
  CloseRearDoor/1(y) -> Data Type Conversion1/1

== system TIA/Baler/SemiAutoCfg Subsystem/CalcTargetSpeed ==
  SwathVolFlowaRate : Inport
  MATLAB Function : MATLAB Function  TreatAsAtomicUnit=on
  Out2 : Outport
  wires:
  SwathVolFlowaRate/1 -> MATLAB Function/1(u)
  MATLAB Function/1(TargetSpeed) -> Out2/1

== system TIA/Baler/SemiAutoCfg Subsystem/RearDoorControl ==
  In1 : Inport
  In2 : Inport  Port=2
  In3 : Inport  Port=3
  In4 : Inport  Port=4
  DoorCmd : Inport  Port=5
  CloseRearDoor : MATLAB Function  TreatAsAtomicUnit=on
  Data Type Conversion1 : DataTypeConversion  OutDataTypeStr=boolean
  OpenRearDoorFunction : MATLAB Function  TreatAsAtomicUnit=on
  Unit Delay : UnitDelay  SampleTime=-1
  Out1 : Outport
  Out2 : Outport  Port=2
  wires:
  CloseRearDoor/1(y) -> Data Type Conversion1/1
  In3/1 -> OpenRearDoorFunction/3(RearObstSr)
  OpenRearDoorFunction/1(Y) -> CloseRearDoor/1(DoorStatus)
  Data Type Conversion1/1 -> Unit Delay/1
  In1/1 -> OpenRearDoorFunction/2(BaleSize)
  In2/1 -> OpenRearDoorFunction/1(StopSignal)
  In4/1 -> CloseRearDoor/2(BaleOutSr)
  DoorCmd/1 -> Out2/1
  Unit Delay/1 -> Out1/1

== system TIA/SwathScanner/Auto_1_Cfg Subsystem/CalcVolFlowRate 1 ==
  CurrentSpeed : Inport
  SwathArea : Inport  Port=2
  MATLAB Function : MATLAB Function  TreatAsAtomicUnit=on
  Out1 : Outport
  wires:
  MATLAB Function/1(y) -> Out1/1
  SwathArea/1 -> MATLAB Function/2(area)
  CurrentSpeed/1 -> MATLAB Function/1(speed)

== system TIA/SwathScanner/Auto_2_Cfg Subsystem/CalcVolFlowRate 1 ==
  CurrentSpeed : Inport
  SwathArea : Inport  Port=2
  MATLAB Function : MATLAB Function  TreatAsAtomicUnit=on
  Out1 : Outport
  wires:
  CurrentSpeed/1 -> MATLAB Function/1(speed)
  SwathArea/1 -> MATLAB Function/2(area)
  MATLAB Function/1(y) -> Out1/1

== system TIA/SwathScanner/Manual_Cfg Subsystem/CalcVolFlowRate 1 ==
  CurrentSpeed : Inport
  SwathArea : Inport  Port=2
  MATLAB Function : MATLAB Function  TreatAsAtomicUnit=on
  Out1 : Outport
  wires:
  MATLAB Function/1(y) -> Out1/1
  SwathArea/1 -> MATLAB Function/2(area)
  CurrentSpeed/1 -> MATLAB Function/1(speed)

== system TIA/SwathScanner/SemiAuto_Cfg Subsystem/CalcVolFlowRate 1 ==
  CurrentSpeed : Inport
  SwathArea : Inport  Port=2
  MATLAB Function : MATLAB Function  TreatAsAtomicUnit=on
  Out1 : Outport
  wires:
  MATLAB Function/1(y) -> Out1/1
  SwathArea/1 -> MATLAB Function/2(area)
  CurrentSpeed/1 -> MATLAB Function/1(speed)

== system TIA/Tractor/Auto_Cfg SubSystem/ValveController ==
  In1 : Inport
  Constant : Constant
  Constant1 : Constant  Value=0
  Data Type Conversion : DataTypeConversion  OutDataTypeStr=boolean
  Switch : Switch  Criteria=u2 ~= 0
  Out1 : Outport
  wires:
  In1/1 -> Switch/2
  Switch/1 -> Data Type Conversion/1
  Constant1/1 -> Switch/3
  Constant/1 -> Switch/1
  Data Type Conversion/1 -> Out1/1

== system TIA/Tractor/ManualCfg SubSystem/ValveController ==
  In1 : Inport
  Constant : Constant
  Constant1 : Constant  Value=0
  Data Type Conversion : DataTypeConversion  OutDataTypeStr=boolean
  Switch : Switch  Criteria=u2 ~= 0
  Out1 : Outport
  wires:
  In1/1 -> Switch/2
  Switch/1 -> Data Type Conversion/1
  Constant1/1 -> Switch/3
  Constant/1 -> Switch/1
  Data Type Conversion/1 -> Out1/1

== system TIA/Tractor/SemiAuto_Cfg SubSystem/ValveController ==
  In1 : Inport
  Constant : Constant
  Constant1 : Constant  Value=0
  Data Type Conversion : DataTypeConversion  OutDataTypeStr=boolean
  Switch : Switch  Criteria=u2 ~= 0
  Out1 : Outport
  wires:
  Data Type Conversion/1 -> Out1/1
  Constant/1 -> Switch/1
  Constant1/1 -> Switch/3
  Switch/1 -> Data Type Conversion/1
  In1/1 -> Switch/2

== matlab function TIA/Baler/AutoCfg_1 SubSystem/CalcTargetSpeed/MATLAB Function ==
  data: u input; TargetSpeed output
function TargetSpeed = fcn(u)

  
TargetSpeed = -.10*u+20;
end

== matlab function TIA/SwathScanner/Manual_Cfg Subsystem/CalcVolFlowRate 1/MATLAB Function ==
  data: speed input; y output; area input
function y = fcn(speed, area)

y = speed*area;
